simulink model "PandO"  (Simulink 7.1)
settings: Solver=ode45  StartTime=0.0  StopTime=10.0  RelTol=1e-3
settings Model: Creator=jagan  LastModifiedBy=jagan

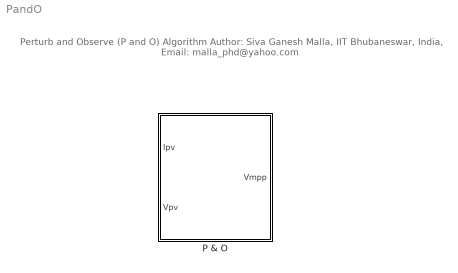
== system PandO ==
  note: Perturb and Observe (P and O) Algorithm
      | Author: Siva Ganesh Malla, IIT Bhubaneswar,
      | India, Email: malla_phd@yahoo.com
  P & O : Subsystem

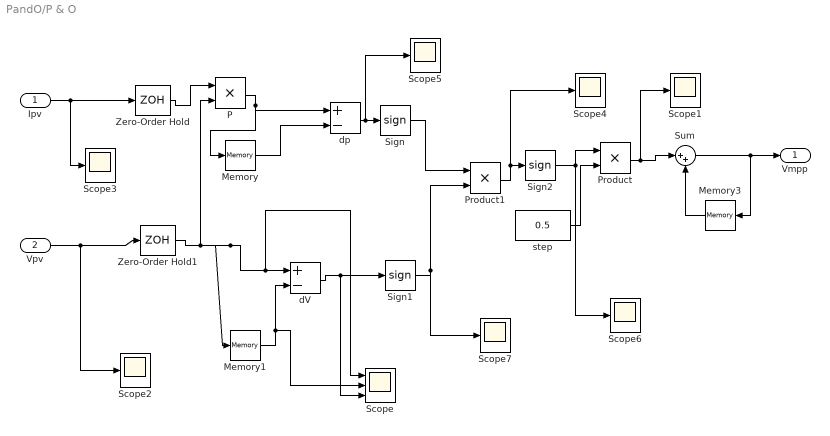
== system PandO/P & O ==
  Ipv : Inport  OutDataType=sfix(16)  OutScaling=2^0
  Vpv : Inport  Port=2  OutDataType=sfix(16)  OutScaling=2^0
  Memory : Memory  InheritSampleTime=on
  Memory1 : Memory  InheritSampleTime=on
  Memory3 : Memory  Orientation=left  InheritSampleTime=on
  P : Product  OutDataType=sfix(16)  OutScaling=2^0  RndMeth=Zero
  Product : Product  OutDataType=sfix(16)  OutScaling=2^0  RndMeth=Zero
  Product1 : Product  OutDataType=sfix(16)  OutScaling=2^0  RndMeth=Zero
  Scope : Scope  NumInputPorts=3
      settings: YMin=29.1717~29.1717~1e-006  YMax=32.2424~32.2424~1.7e-005
  Scope{1..7} (7 alike) : Scope
      Scope1 settings: YMin=-0.0005  YMax=0.0005  SaveName=ScopeData34
      Scope2 settings: YMin=-11  YMax=10  SaveName=ScopeData35
      Scope3 settings: YMin=-11  YMax=10  SaveName=ScopeData36
      Scope4 settings: YMin=-11  YMax=10  SaveName=ScopeData37
      Scope5 settings: YMin=-11  YMax=10
      Scope6 settings: YMin=-11  YMax=10  SaveName=ScopeData38
      Scope7 settings: YMin=-11  YMax=10  SaveName=ScopeData39
  Sign : Signum
  Sign1 : Signum
  Sign2 : Signum
  Sum : Sum  Inputs=|++  OutDataType=sfix(16)  OutScaling=2^0
  Zero-Order Hold : ZeroOrderHold  SampleTime=0.002
  Zero-Order Hold1 : ZeroOrderHold  SampleTime=0.002
  dV : Sum  Inputs=+-  OutDataType=sfix(16)  OutScaling=2^-10
  dp : Sum  Inputs=+-  OutDataType=sfix(16)  OutScaling=2^-10
  step : Constant  Value=0.5  OutDataType=sfix(16)  OutScaling=2^0
  Vmpp : Outport  OutDataType=sfix(16)  OutScaling=2^0
  wires:
  Memory1/1 -> dV/2, Scope/2
  Memory/1 -> dp/2
  Vpv/1 -> Zero-Order Hold1/1, Scope2/1
  dV/1 -> Sign1/1, Scope/3
  step/1 -> Product/2
  Product/1 -> Sum/1, Scope1/1
  Sign/1 -> Product1/1
  Sign1/1 -> Product1/2, Scope7/1
  Product1/1 -> Sign2/1, Scope4/1
  Ipv/1 -> Zero-Order Hold/1, Scope3/1
  Zero-Order Hold1/1 -> P/2, Memory1/1, dV/1, Scope/1
  Zero-Order Hold/1 -> P/1
  P/1 -> Memory/1, dp/1
  dp/1 -> Sign/1, Scope5/1
  Sign2/1 -> Product/1, Scope6/1
  Sum/1 -> Memory3/1, Vmpp/1
  Memory3/1 -> Sum/2
